simulink model "model2"  (R2021b)
settings: Solver=VariableStepAuto  StartTime=0.0  StopTime=30  RelTol=0.001
settings Model: Creator=AMY  LastModifiedBy=AMY

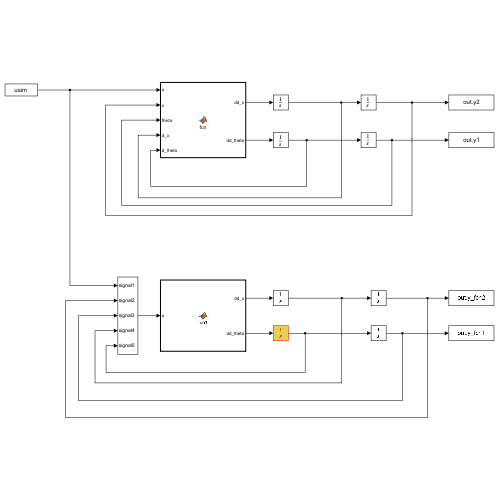
[thumbnail: Simulink's stored preview of the top-level diagram]
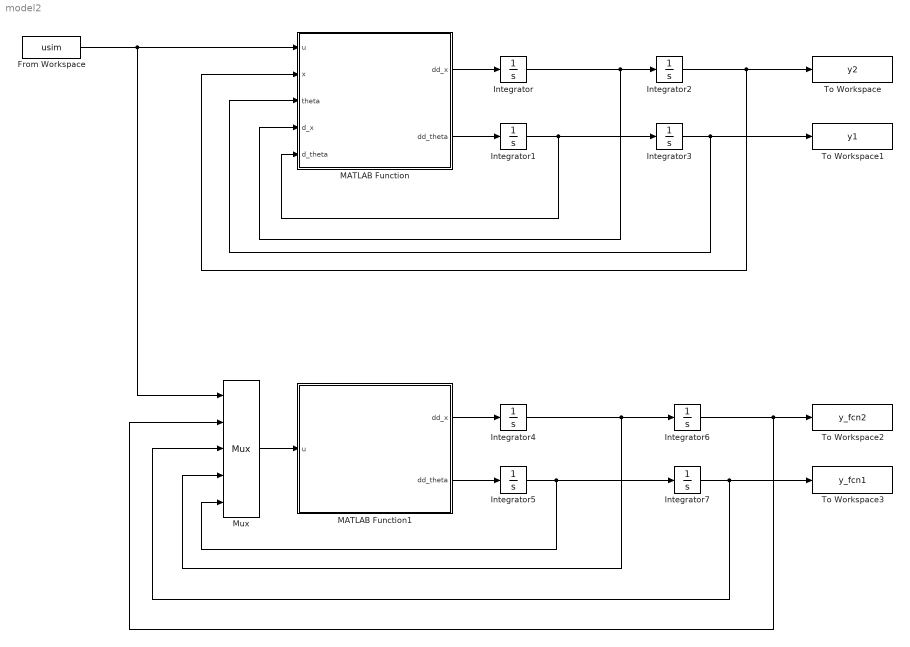
== system model2 ==
  From Workspace : FromWorkspace  VariableName=usim
  Integrator{,1..7} (8 alike) : Integrator
  MATLAB Function : MATLAB Function  TreatAsAtomicUnit=on
  MATLAB Function1 : MATLAB Function  TreatAsAtomicUnit=on
  Mux : Mux  Inputs=5
      settings: DisplayOption=signals
  To Workspace : ToWorkspace  VariableName=y2  SaveFormat=Timeseries  SampleTime=-1
      settings: Save2DSignal=2-D array (concatenate along first dimension)
  To Workspace1 : ToWorkspace  VariableName=y1  SaveFormat=Timeseries  SampleTime=-1
      settings: Save2DSignal=2-D array (concatenate along first dimension)
  To Workspace2 : ToWorkspace  VariableName=y_fcn2  SaveFormat=Timeseries  SampleTime=-1
      settings: Save2DSignal=2-D array (concatenate along first dimension)
  To Workspace3 : ToWorkspace  VariableName=y_fcn1  SaveFormat=Timeseries  SampleTime=-1
      settings: Save2DSignal=2-D array (concatenate along first dimension)
  wires:
  From Workspace/1 -> Mux/1, MATLAB Function/1(u)
  MATLAB Function/1(dd_x) -> Integrator/1
  MATLAB Function/2(dd_theta) -> Integrator1/1
  Integrator/1 -> MATLAB Function/4(d_x), Integrator2/1
  Integrator1/1 -> Integrator3/1, MATLAB Function/5(d_theta)
  Integrator3/1 -> To Workspace1/1, MATLAB Function/3(theta)
  Integrator2/1 -> To Workspace/1, MATLAB Function/2(x)
  Mux/1 -> MATLAB Function1/1(u)
  MATLAB Function1/1(dd_x) -> Integrator4/1
  Integrator4/1 -> Integrator6/1, Mux/4
  MATLAB Function1/2(dd_theta) -> Integrator5/1
  Integrator5/1 -> Integrator7/1, Mux/5
  Integrator7/1 -> To Workspace3/1, Mux/3
  Integrator6/1 -> Mux/2, To Workspace2/1

== matlab function model2/MATLAB Function1 ==
  data: u input; dd_x output; dd_theta output
function [dd_x, dd_theta] = fcn1(u)

    m = 1.5;          %Masa corpului
    g = 9.81;         %Acceleratia gravitationala
    zeta = 0.6;       %Coeficient de amortizare
    k = 1.5;          %Constanta elastica
    l0 = 0.5;         %Lungimea initiala a resortului
    
    %Ecuatiile
    dd_x = (l0+u(2))*(u(5))*(u(5)) - (k/m)*u(2) + g*cos(u(3)) - zeta*u(4);
    dd_theta = -(g/(l0+u(2))*sin(u(3)))-(2*u(4)/(l0+u(2)))*u(5) - zeta*u(5) + 1/(m*(l0+u(2))*(l0+u(2)))*u(1);

end

== matlab function model2/MATLAB Function ==
  data: dd_x output; u input; dd_theta output; x input; theta input; d_x input; d_theta input
function [dd_x, dd_theta] = fcn(u, x, theta,  d_x, d_theta)

    m = 1.5;          %Masa corpului
    g = 9.81;         %Acceleratia gravitationala
    zeta = 0.6;      %Coeficient de amortizare
    k = 1.5;          %Constanta elastica
    l0 = 0.5;         %Lungimea initiala a resortului
    
    %Ecuatiile
    dd_x = (l0+x)*(d_theta)*(d_theta) - (k/m)*x + g*cos(theta) - zeta*d_x;
    dd_theta = -(g/(l0+x)*sin(theta))-(2*d_x/(l0+x))*d_theta - zeta*d_theta + 1/(m*(l0+x)*(l0+x))*u;

end
